simulink library "Brakes_ABS_4_Channel"  (R2019b)
settings: Solver=VariableStepAuto  StartTime=0.0  StopTime=10.0  RelTol=1e-3
undefined symbols (not defined in the file): Brakes
libraries: fl_lib x31, nesl_utility x18, sh_lib x9, sdl_lib x4, sm_car_lib x4
(part 1 of 2)
Description:
  | Component of Simscape Vehicle Templates Library
  | 
  | Copyright 2018-2020 The MathWorks, Inc.
settings Model: Creator=smiller  LastModifiedBy=smiller
settings DataIOCC: ReturnWorkspaceOutputs=off
settings DebuggingCC: ArithmeticOperatorsInVariantConditions=warning
settings SFSimCC: CustomCodeUndefinedFunction=UseInterfaceOnly

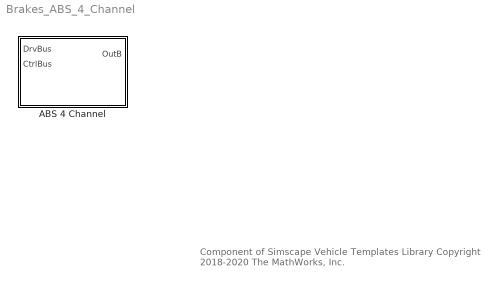
== system Brakes_ABS_4_Channel ==
  note: Component of Simscape Vehicle Templates Library
      | Copyright 2018-2020 The MathWorks, Inc.
  ABS 4 Channel : Subsystem  Tag=PublishSubsystem  VariantControl=ABS_4_Channel  mask(Four Channel ABS){d_caliper_bore_f=Brakes.Front.Caliper.lCylinderDiameter.Value, d_caliper_bore_r=Brakes.Rear.Caliper.lCylinderDiameter.Value, brk_pad_rad_fa=Brakes.Front.DiscAndPad.lMeanRadius.Value, brk_pad_rad_ra=Brakes.Rear.DiscAndPad.lMeanRadius.Value, brk_cyl_bore_fa=Brakes.Front.Caliper.lCylinderDiameter.Value, brk_cyl_bore_ra=Brakes.Rear.Caliper.lCylinderDiameter.Value, brk_n_pads_fa=Brakes.Front.DiscAndPad.NPads.Value, brk_n_pads_ra=Brakes.Rear.DiscAndPad.NPads.Value, brk_mu_static_fa=Brakes.Front.DiscAndPad.rMuStatic.Value, brk_mu_static_ra=Brakes.Rear.DiscAndPad.rMuStatic.Value, brk_mu_kin_fa=Brakes.Front.DiscAndPad.rMuKinetic.Value, brk_mu_kin_ra=Brakes.Rear.DiscAndPad.rMuKinetic.Value, brk_trans_vel_fa=Brakes.Front.DiscAndPad.nTransition.Value, brk_trans_vel_ra=Brakes.Rear.DiscAndPad.nTransition.Value, brk_visc_coef_fa=Brakes.Front.DiscAndPad.dViscous.Value, brk_visc_coef_ra=Brakes.Rear.DiscAndPad.dViscous.Value, spr_rate=Brakes.Front.ValveApply.kSpring.Value, D=Brakes.Front.ValveApply.bDamper.Value, area_max_apply=Brakes.Front.ValveApply.AMax.Value, open_max_apply=Brakes.Front.ValveApply.xMax.Value, area_max_rel=Brakes.Front.ValveRelease.AMax.Value, open_max_rel=Brakes.Front.ValveRelease.xMax.Value, p_max_f=Brakes.Front.Caliper.pMax.Value, p_max_r=Brakes.Rear.Caliper.pMax.Value, brkTs=Brakes.Front.ValveApply.fValveTime.Value}
      mask prompts: spr_rate "Spring Rate (N/m)"; D "Damping coefficient"; area_max_apply "Max Area Apply Valve (m^2)"; open_max_apply "Max Opening Apply Valve (m)"; area_max_rel "Max Area Release Valve (m^2)"; open_max_rel "Max Opening Release Valve (m)"; p_max_f "Max Master Cylinder Pressure Front (bar)"; p_max_r "Max Master Cylinder Pressure Rear (bar)"; brkTs "Filter time constant"
      mask init:
      | pist_area_pist_f = pi*d_caliper_bore_f^2/4;
      | pist_area_pist_r = pi*d_caliper_bore_r^2/4;
      mask TypeOptions brk_pad_rad_fa:
      | Disc
      | Brake
      | FL/r_mean | Disc
      | Brake
      | FR/r_mean
      mask TypeOptions brk_pad_rad_ra:
      | Disc
      | Brake
      | RL/r_mean | Disc
      | Brake
      | RR/r_mean
      mask TypeOptions brk_cyl_bore_fa:
      | Disc
      | Brake
      | FL/bore | Disc
      | Brake
      | FR/bore
      mask TypeOptions brk_cyl_bore_ra:
      | Disc
      | Brake
      | RL/bore | Disc
      | Brake
      | RR/bore
      mask TypeOptions brk_n_pads_fa:
      | Disc
      | Brake
      | FL/n_pads | Disc
      | Brake
      | FR/n_pads
      mask TypeOptions brk_n_pads_ra:
      | Disc
      | Brake
      | RL/n_pads | Disc
      | Brake
      | RR/n_pads
      mask TypeOptions brk_mu_static_fa:
      | Disc
      | Brake
      | FL/mu_static | Disc
      | Brake
      | FR/mu_static
      mask TypeOptions brk_mu_static_ra:
      | Disc
      | Brake
      | RL/mu_static | Disc
      | Brake
      | RR/mu_static
      mask TypeOptions brk_mu_kin_fa:
      | Disc
      | Brake
      | FL/mu_coulomb | Disc
      | Brake
      | FR/mu_coulomb
      mask TypeOptions brk_mu_kin_ra:
      | Disc
      | Brake
      | RL/mu_coulomb | Disc
      | Brake
      | RR/mu_coulomb
      mask TypeOptions brk_trans_vel_fa:
      | Disc
      | Brake
      | FL/brkwy_vel | Disc
      | Brake
      | FR/brkwy_vel
      mask TypeOptions brk_trans_vel_ra:
      | Disc
      | Brake
      | RL/brkwy_vel | Disc
      | Brake
      | RR/brkwy_vel
      mask TypeOptions brk_visc_coef_fa:
      | Disc
      | Brake
      | FL/visc_coef
      mask TypeOptions brk_visc_coef_ra:
      | Disc
      | Brake
      | RL/visc_coef | Disc
      | Brake
      | RR/visc_coef
      mask TypeOptions spr_rate: Valves/spr_rate
      mask TypeOptions D: Valves/D
      mask TypeOptions area_max_apply: Valves/area_max_apply
      mask TypeOptions open_max_apply: Valves/open_max_apply
      mask TypeOptions area_max_rel: Valves/area_max_rel
      mask TypeOptions open_max_rel: Valves/open_max_rel
      mask TypeOptions p_max_f: Valves/p_max_f
      mask TypeOptions p_max_r: Valves/p_max_r
      mask TypeOptions brkTs: Valves/brkTs
      mask DialogControl Container10 Prompt: Geometry
      mask DialogControl cont_brk_geom Prompt: Geometry
      mask DialogControl text_brakes_fa Prompt: Front Susp.
      mask DialogControl text_brakes_ra Prompt: Rear Susp.
      mask DialogControl text_caliper_bore Prompt: Caliper Bore (m)
      mask DialogControl text_brakes_pad_rad Prompt: Mean Pad Radius (m)
      mask DialogControl text_brakes_cyl_bore Prompt: Cylinder Bore (m)
      mask DialogControl text_brakes_n_pads Prompt: Number of pads
      mask DialogControl Container9 Prompt: Friction
      mask DialogControl cont_brk_frict Prompt: Friction
      mask DialogControl text_brakes_mu_static Prompt: Static Coeff. (0-1)
      mask DialogControl text_brakes_mu_kin Prompt: Kinetic Coeff. (0-1)
      mask DialogControl text_brakes_trans_vel Prompt: Trans. Velocity (rad/s)
      mask DialogControl text_brakes_visc_coef Prompt: Viscous (N*m/(rad/s))
      mask DialogControl cont_valves Prompt: Valves
      mask Display: image('sm_car_vehicle_brakes_abs_IMAGE.png');

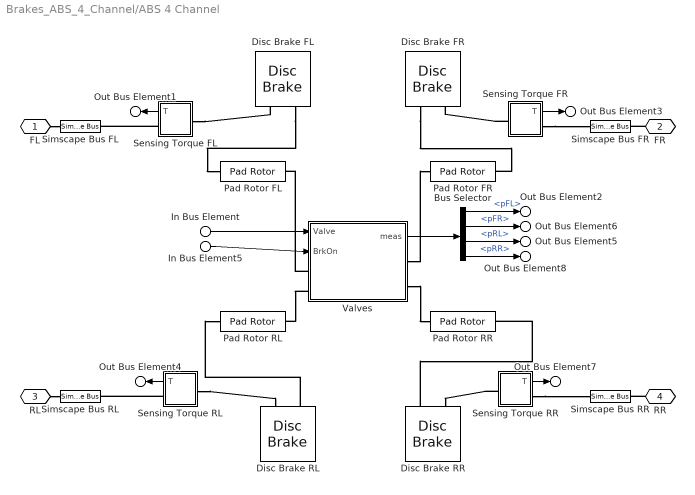
== system Brakes_ABS_4_Channel/ABS 4 Channel ==
  In Bus Element5 : Inport  PortName=DrvBus  Element=rBrakePedal
  In Bus Element : Inport  Port=2  PortName=CtrlBus  Element=Valves
  Bus Selector : BusSelector  OutputSignals=pFL,pFR,pRL,pRR
  Disc Brake FL : sdl_lib/Brakes & Detents/Rotational/Disc Brake  r_mean=brk_pad_rad_fa m  bore=brk_cyl_bore_fa m  n_pads=brk_n_pads_fa  thermal_port=simscape.enum.thermaleffects.omit  mu_static=brk_mu_static_fa  mu_coulomb=brk_mu_kin_fa  temperature_TLU=[280, 300, 320] K  mu_static_TLU=[.9, .8, .7]  mu_coulomb_TLU=[.8, .7, .6]  thermal_mass=50 kJ/K  brkwy_vel=brk_trans_vel_fa rad/s  visc_coef=brk_visc_coef_fa N*m/(rad/s)  temperature_specify=off  temperature_priority=High  temperature=300 K  temperature_nominal_specify=off  temperature_nominal_unit=K  temperature_nominal_value=1
      settings: SourceProductName=Simscape Driveline  SourceProductBaseCode=LD
  Disc Brake FR : sdl_lib/Brakes & Detents/Rotational/Disc Brake  r_mean=brk_pad_rad_fa m  bore=brk_cyl_bore_fa m  n_pads=brk_n_pads_fa  thermal_port=simscape.enum.thermaleffects.omit  mu_static=brk_mu_static_fa  mu_coulomb=brk_mu_kin_fa  temperature_TLU=[280, 300, 320] K  mu_static_TLU=[.9, .8, .7]  mu_coulomb_TLU=[.8, .7, .6]  thermal_mass=50 kJ/K  brkwy_vel=brk_trans_vel_fa rad/s  visc_coef=.001 N*m/(rad/s)  temperature_specify=off  temperature_priority=High  temperature=300 K  temperature_nominal_specify=off  temperature_nominal_unit=K  temperature_nominal_value=1
      settings: SourceProductName=Simscape Driveline  SourceProductBaseCode=LD
  Disc Brake RL : sdl_lib/Brakes & Detents/Rotational/Disc Brake  r_mean=brk_pad_rad_ra m  bore=brk_cyl_bore_ra m  n_pads=brk_n_pads_ra  thermal_port=simscape.enum.thermaleffects.omit  mu_static=brk_mu_static_ra  mu_coulomb=brk_mu_kin_ra  temperature_TLU=[280, 300, 320] K  mu_static_TLU=[.9, .8, .7]  mu_coulomb_TLU=[.8, .7, .6]  thermal_mass=50 kJ/K  brkwy_vel=brk_trans_vel_ra rad/s  visc_coef=brk_visc_coef_ra N*m/(rad/s)  temperature_specify=off  temperature_priority=High  temperature=300 K  temperature_nominal_specify=off  temperature_nominal_unit=K  temperature_nominal_value=1
      settings: SourceProductName=Simscape Driveline  SourceProductBaseCode=LD
  Disc Brake RR : sdl_lib/Brakes & Detents/Rotational/Disc Brake  r_mean=brk_pad_rad_ra m  bore=brk_cyl_bore_ra m  n_pads=brk_n_pads_ra  thermal_port=simscape.enum.thermaleffects.omit  mu_static=brk_mu_static_ra  mu_coulomb=brk_mu_kin_ra  temperature_TLU=[280, 300, 320] K  mu_static_TLU=[.9, .8, .7]  mu_coulomb_TLU=[.8, .7, .6]  thermal_mass=50 kJ/K  brkwy_vel=brk_trans_vel_ra rad/s  visc_coef=brk_visc_coef_ra N*m/(rad/s)  temperature_specify=off  temperature_priority=High  temperature=300 K  temperature_nominal_specify=off  temperature_nominal_unit=K  temperature_nominal_value=1
      settings: SourceProductName=Simscape Driveline  SourceProductBaseCode=LD
  Pad Rotor FL : sm_car_lib/Brakes/Pad Rotor  d_caliper_piston_f=d_caliper_bore_f
  Pad Rotor FR : sm_car_lib/Brakes/Pad Rotor  d_caliper_piston_f=d_caliper_bore_f
  Pad Rotor RL : sm_car_lib/Brakes/Pad Rotor  d_caliper_piston_f=d_caliper_bore_r
  Pad Rotor RR : sm_car_lib/Brakes/Pad Rotor  d_caliper_piston_f=d_caliper_bore_r
  Sensing Torque FL : Subsystem
  Sensing Torque FR : Subsystem
  Sensing Torque RL : Subsystem
  Sensing Torque RR : Subsystem
  Simscape Bus FL : SimscapeBus  HierarchyStrings=Axle1D
  Simscape Bus FR : SimscapeBus  HierarchyStrings=Axle1D
  Simscape Bus RL : SimscapeBus  HierarchyStrings=Axle1D
  Simscape Bus RR : SimscapeBus  HierarchyStrings=Axle1D
  Valves : Subsystem  VariantControl=Valves  mask{brkTs=brkTs, p_max_f=p_max_f, p_max_r=p_max_r, spr_rate=spr_rate, D=D, area_max_apply=area_max_apply, open_max_apply=open_max_apply, area_max_rel=area_max_rel, open_max_rel=open_max_rel}
      mask prompts: brkTs "Filter time constant"; p_max_f "Max Pressure Front (bar)"; p_max_r "Max Pressure Rear (bar)"; spr_rate "Spring Rate (N/m)"; D "Damping coefficient"; area_max_apply "Max Area Apply Valve (m^2)"; open_max_apply "Max Opening Apply Valve (m)"; area_max_rel "Max Area Release Valve (m^2)"; open_max_rel "Max Opening Release Valve (m)"
      mask TypeOptions brkTs:
      | Valves FL/Actuator
      | Dynamics/b | Valves FR/Actuator
      | Dynamics/b | Valves RL/Actuator
      | Dynamics/b | Valves RR/Actuator
      | Dynamics/b
      mask TypeOptions p_max_f: MC Pressure F/Value
      mask TypeOptions p_max_r: MC Pressure R/Value
      mask TypeOptions spr_rate: Return Spring FL/Spring/spr_rate | Return Spring FR/Spring/spr_rate | Return Spring RL/Spring/spr_rate | Return Spring RR/Spring/spr_rate
      mask TypeOptions D: Return Spring FL/Damper/D | Return Spring FR/Damper/D | Return Spring RL/Damper/D | Return Spring RR/Damper/D
  FL : PMIOPort  Side=Left
  FR : PMIOPort  Port=2  Side=Right
  RL : PMIOPort  Port=3  Side=Left
  RR : PMIOPort  Port=4  Side=Right
  Out Bus Element1 : Outport  VectorParamsAs1DForOutWhenUnconnected=off  PortName=OutB  Element=MBrakeFL
  Out Bus Element3 : Outport  VectorParamsAs1DForOutWhenUnconnected=off  PortName=OutB  Element=MBrakeFR
  Out Bus Element4 : Outport  VectorParamsAs1DForOutWhenUnconnected=off  PortName=OutB  Element=MBrakeRL
  Out Bus Element7 : Outport  VectorParamsAs1DForOutWhenUnconnected=off  PortName=OutB  Element=MBrakeRR
  Out Bus Element2 : Outport  VectorParamsAs1DForOutWhenUnconnected=off  PortName=OutB  Element=pBrakeFL
  Out Bus Element6 : Outport  VectorParamsAs1DForOutWhenUnconnected=off  PortName=OutB  Element=pBrakeFR
  Out Bus Element5 : Outport  VectorParamsAs1DForOutWhenUnconnected=off  PortName=OutB  Element=pBrakeRL
  Out Bus Element8 : Outport  VectorParamsAs1DForOutWhenUnconnected=off  PortName=OutB  Element=pBrakeRR
  wires:
  Sensing Torque FL/1(T) -> Out Bus Element1/1
  Bus Selector/4 -> Out Bus Element8/1  "<pRR>"
  Sensing Torque FR/1(T) -> Out Bus Element3/1
  Sensing Torque RR/1(T) -> Out Bus Element7/1
  Bus Selector/2 -> Out Bus Element6/1  "<pFR>"
  Bus Selector/1 -> Out Bus Element2/1  "<pFL>"
  Sensing Torque RL/1(T) -> Out Bus Element4/1
  Bus Selector/3 -> Out Bus Element5/1  "<pRL>"
  Valves/1(meas) -> Bus Selector/1
  In Bus Element/1 -> Valves/1(Valve)
  In Bus Element5/1 -> Valves/2(BrkOn)
  connections:
  Sensing Torque RL/RConn1 -- Simscape Bus RL/LConn1
  Valves/LConn2 -- Pad Rotor RL/RConn1
  Disc Brake FR/LConn1 -- Pad Rotor FR/LConn1
  Sensing Torque FR/LConn1 -- Disc Brake FR/LConn2
  Disc Brake RR/LConn1 -- Pad Rotor RR/LConn1
  Valves/RConn2 -- Pad Rotor RR/RConn1
  RL/RConn1 -- Simscape Bus RL/RConn1
  Sensing Torque RR/LConn1 -- Disc Brake RR/LConn2
  Sensing Torque FR/RConn1 -- Simscape Bus FR/LConn1
  Disc Brake RL/LConn1 -- Pad Rotor RL/LConn1
  Sensing Torque RR/RConn1 -- Simscape Bus RR/LConn1
  Sensing Torque FL/RConn1 -- Simscape Bus FL/LConn1
  Sensing Torque FL/LConn1 -- Disc Brake FL/LConn2
  RR/RConn1 -- Simscape Bus RR/RConn1
  FR/RConn1 -- Simscape Bus FR/RConn1
  Sensing Torque RL/LConn1 -- Disc Brake RL/LConn2
  Valves/LConn1 -- Pad Rotor FL/RConn1
  Disc Brake FL/LConn1 -- Pad Rotor FL/LConn1
  FL/RConn1 -- Simscape Bus FL/RConn1
  Valves/RConn1 -- Pad Rotor FR/RConn1

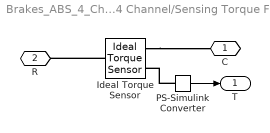
== system Brakes_ABS_4_Channel/ABS 4 Channel/Sensing Torque FL ==
  Ideal Torque Sensor : fl_lib/Mechanical/Mechanical Sensors/Ideal Torque Sensor
  PS-Simulink Converter : nesl_utility/PS-Simulink Converter  PhysicalDomain=network_engine_domain  SubClassName=ps_output  LeftPortType=input  RightPortType=output  PseudoPeriodic=off  Frequencies=[]  Unit=N*m  AffineConversion=off
  C : PMIOPort  Side=Right
  R : PMIOPort  Port=2  Side=Left
  T : Outport  VectorParamsAs1DForOutWhenUnconnected=off
  wires:
  PS-Simulink Converter/1 -> T/1
  connections:
  Ideal Torque Sensor/LConn1 -- R/RConn1
  Ideal Torque Sensor/RConn1 -- C/RConn1
  PS-Simulink Converter/LConn1 -- Ideal Torque Sensor/RConn2

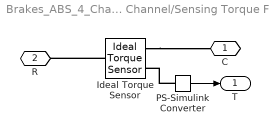
== system Brakes_ABS_4_Channel/ABS 4 Channel/Sensing Torque FR ==
  Ideal Torque Sensor : fl_lib/Mechanical/Mechanical Sensors/Ideal Torque Sensor
  PS-Simulink Converter : nesl_utility/PS-Simulink Converter  PhysicalDomain=network_engine_domain  SubClassName=ps_output  LeftPortType=input  RightPortType=output  PseudoPeriodic=off  Frequencies=[]  Unit=N*m  AffineConversion=off
  C : PMIOPort  Side=Right
  R : PMIOPort  Port=2  Side=Left
  T : Outport  VectorParamsAs1DForOutWhenUnconnected=off
  wires:
  PS-Simulink Converter/1 -> T/1
  connections:
  Ideal Torque Sensor/LConn1 -- R/RConn1
  Ideal Torque Sensor/RConn1 -- C/RConn1
  PS-Simulink Converter/LConn1 -- Ideal Torque Sensor/RConn2

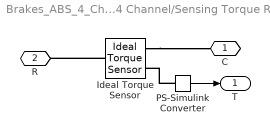
== system Brakes_ABS_4_Channel/ABS 4 Channel/Sensing Torque RL ==
  Ideal Torque Sensor : fl_lib/Mechanical/Mechanical Sensors/Ideal Torque Sensor
  PS-Simulink Converter : nesl_utility/PS-Simulink Converter  PhysicalDomain=network_engine_domain  SubClassName=ps_output  LeftPortType=input  RightPortType=output  PseudoPeriodic=off  Frequencies=[]  Unit=N*m  AffineConversion=off
  C : PMIOPort  Side=Right
  R : PMIOPort  Port=2  Side=Left
  T : Outport  VectorParamsAs1DForOutWhenUnconnected=off
  wires:
  PS-Simulink Converter/1 -> T/1
  connections:
  PS-Simulink Converter/LConn1 -- Ideal Torque Sensor/RConn2
  Ideal Torque Sensor/RConn1 -- C/RConn1
  Ideal Torque Sensor/LConn1 -- R/RConn1

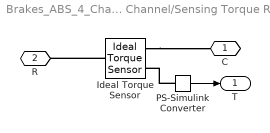
== system Brakes_ABS_4_Channel/ABS 4 Channel/Sensing Torque RR ==
  Ideal Torque Sensor : fl_lib/Mechanical/Mechanical Sensors/Ideal Torque Sensor
  PS-Simulink Converter : nesl_utility/PS-Simulink Converter  PhysicalDomain=network_engine_domain  SubClassName=ps_output  LeftPortType=input  RightPortType=output  PseudoPeriodic=off  Frequencies=[]  Unit=N*m  AffineConversion=off
  C : PMIOPort  Side=Right
  R : PMIOPort  Port=2  Side=Left
  T : Outport  VectorParamsAs1DForOutWhenUnconnected=off
  wires:
  PS-Simulink Converter/1 -> T/1
  connections:
  PS-Simulink Converter/LConn1 -- Ideal Torque Sensor/RConn2
  Ideal Torque Sensor/RConn1 -- C/RConn1
  Ideal Torque Sensor/LConn1 -- R/RConn1

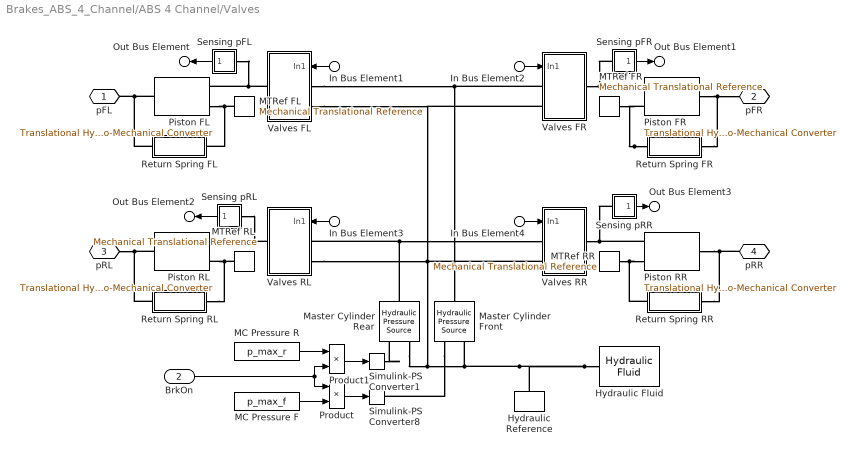
== system Brakes_ABS_4_Channel/ABS 4 Channel/Valves ==
  In Bus Element1 : Inport  PortName=Valve  Element=FL
  In Bus Element2 : Inport  PortName=Valve  Element=FR
  In Bus Element3 : Inport  PortName=Valve  Element=RL
  In Bus Element4 : Inport  PortName=Valve  Element=RR
  BrkOn : Inport  Port=2
  Hydraulic Fluid : sh_lib/Hydraulic Utilities/Hydraulic Fluid  DataSource=1  SelFluid=17  SysTemp=60  TrapAir=0.005  ViscDerFactor=1  range_error=2
      settings: SourceProductName=Simscape Fluids
  Hydraulic Reference : fl_lib/Hydraulic/Hydraulic Elements/Hydraulic Reference
      settings: SourceProductName=Simscape
  MC Pressure F : Constant  Value=p_max_f
  MC Pressure R : Constant  Value=p_max_r
  MTRef FL : fl_lib/Mechanical/Translational Elements/Mechanical Translational Reference
  MTRef FR : fl_lib/Mechanical/Translational Elements/Mechanical Translational Reference
  MTRef RL : fl_lib/Mechanical/Translational Elements/Mechanical Translational Reference
  MTRef RR : fl_lib/Mechanical/Translational Elements/Mechanical Translational Reference
  Master Cylinder Front : fl_lib/Hydraulic/Hydraulic Sources/Hydraulic Pressure Source
      settings: SourceProductName=Simscape  SourceProductBaseCode=SS  InternalSimscapePortConfiguration="{\"Bottom\":[],\"Left\":[{\"id\":\"P\",\"label\":\"P\",\"type\":\"foundation.hydraulic.hydraulic\"}],\"Right\":[{\"id\":\"S\",\"label\":\"S\",\"type\":\"input\"},{\"id\":\"T\",\"label\":\"T\",\"type\":\"foundation.hydraulic.hydraulic\"}],\"Top\":[]}"
  Master Cylinder Rear : fl_lib/Hydraulic/Hydraulic Sources/Hydraulic Pressure Source
      settings: SourceProductName=Simscape  SourceProductBaseCode=SS  InternalSimscapePortConfiguration="{\"Bottom\":[],\"Left\":[{\"id\":\"P\",\"label\":\"P\",\"type\":\"foundation.hydraulic.hydraulic\"}],\"Right\":[{\"id\":\"S\",\"label\":\"S\",\"type\":\"input\"},{\"id\":\"T\",\"label\":\"T\",\"type\":\"foundation.hydraulic.hydraulic\"}],\"Top\":[]}"
  Piston FL : fl_lib/Hydraulic/Hydraulic Elements/Translational Hydro-Mechanical Converter  area=pist_area_pist_f m^2  or=1  compressibility=1  init_pos=0 m  V_dead=1e-4 m^3  k_sh=1.4  initial_pressure=0 Pa
      settings: SourceProductName=Simscape  SourceProductBaseCode=SS  InternalSimscapePortConfiguration="{\"Bottom\":[],\"Left\":[{\"id\":\"C\",\"label\":\"C\",\"type\":\"foundation.mechanical.translational.translational\"},{\"id\":\"A\",\"label\":\"A\",\"type\":\"foundation.hydraulic.hydraulic\"}],\"Right\":[{\"id\":\"R\",\"label\":\"R\",\"type\":\"foundation.mechanical.translational.translational\"}],\"Top\":[]}"
  Piston FR : fl_lib/Hydraulic/Hydraulic Elements/Translational Hydro-Mechanical Converter  area=pist_area_pist_f m^2  or=1  compressibility=1  init_pos=0 m  V_dead=1e-4 m^3  k_sh=1.4  initial_pressure=0 Pa
      settings: SourceProductName=Simscape  SourceProductBaseCode=SS  InternalSimscapePortConfiguration="{\"Bottom\":[],\"Left\":[{\"id\":\"C\",\"label\":\"C\",\"type\":\"foundation.mechanical.translational.translational\"},{\"id\":\"A\",\"label\":\"A\",\"type\":\"foundation.hydraulic.hydraulic\"}],\"Right\":[{\"id\":\"R\",\"label\":\"R\",\"type\":\"foundation.mechanical.translational.translational\"}],\"Top\":[]}"
  Piston RL : fl_lib/Hydraulic/Hydraulic Elements/Translational Hydro-Mechanical Converter  area=pist_area_pist_r m^2  or=1  compressibility=1  init_pos=0 m  V_dead=1e-4 m^3  k_sh=1.4  initial_pressure=0 Pa
      settings: SourceProductName=Simscape  SourceProductBaseCode=SS  InternalSimscapePortConfiguration="{\"Bottom\":[],\"Left\":[{\"id\":\"C\",\"label\":\"C\",\"type\":\"foundation.mechanical.translational.translational\"},{\"id\":\"A\",\"label\":\"A\",\"type\":\"foundation.hydraulic.hydraulic\"}],\"Right\":[{\"id\":\"R\",\"label\":\"R\",\"type\":\"foundation.mechanical.translational.translational\"}],\"Top\":[]}"
  Piston RR : fl_lib/Hydraulic/Hydraulic Elements/Translational Hydro-Mechanical Converter  area=pist_area_pist_r m^2  or=1  compressibility=1  init_pos=0 m  V_dead=1e-4 m^3  k_sh=1.4  initial_pressure=0 Pa
      settings: SourceProductName=Simscape  SourceProductBaseCode=SS  InternalSimscapePortConfiguration="{\"Bottom\":[],\"Left\":[{\"id\":\"C\",\"label\":\"C\",\"type\":\"foundation.mechanical.translational.translational\"},{\"id\":\"A\",\"label\":\"A\",\"type\":\"foundation.hydraulic.hydraulic\"}],\"Right\":[{\"id\":\"R\",\"label\":\"R\",\"type\":\"foundation.mechanical.translational.translational\"}],\"Top\":[]}"
  Product : Product
  Product1 : Product
  Return Spring FL : Subsystem
  Return Spring FR : Subsystem
  Return Spring RL : Subsystem
  Return Spring RR : Subsystem
  Sensing pFL : Subsystem
  Sensing pFR : Subsystem
  Sensing pRL : Subsystem
  Sensing pRR : Subsystem
  Simulink-PS Converter1 : nesl_utility/Simulink-PS Converter  PhysicalDomain=network_engine_domain  SubClassName=ps_input  LeftPortType=input  RightPortType=output  PseudoPeriodic=off  Frequencies=[]  NoiseDistribution=none  NoiseParameters=[]  Unit=bar  AffineConversion=off  FilteringAndDerivatives=provide  SimscapeFilterOrder=1  InputFilterTimeConstant=0.001  UdotUserProvided=0
  Simulink-PS Converter8 : nesl_utility/Simulink-PS Converter  PhysicalDomain=network_engine_domain  SubClassName=ps_input  LeftPortType=input  RightPortType=output  PseudoPeriodic=off  Frequencies=[]  NoiseDistribution=none  NoiseParameters=[]  Unit=bar  AffineConversion=off  FilteringAndDerivatives=provide  SimscapeFilterOrder=1  InputFilterTimeConstant=0.001  UdotUserProvided=0
  Valves FL : Subsystem
  Valves FR : Subsystem
  Valves RL : Subsystem
  Valves RR : Subsystem
  pFL : PMIOPort  Side=Left
  pFR : PMIOPort  Port=2  Side=Right
  pRL : PMIOPort  Port=3  Side=Left
  pRR : PMIOPort  Port=4  Side=Right
  Out Bus Element : Outport  VectorParamsAs1DForOutWhenUnconnected=off  PortName=meas  Element=pFL
  Out Bus Element1 : Outport  VectorParamsAs1DForOutWhenUnconnected=off  PortName=meas  Element=pFR
  Out Bus Element2 : Outport  VectorParamsAs1DForOutWhenUnconnected=off  PortName=meas  Element=pRL
  Out Bus Element3 : Outport  VectorParamsAs1DForOutWhenUnconnected=off  PortName=meas  Element=pRR
  wires:
  Product/1 -> Simulink-PS Converter8/1
  BrkOn/1 -> Product/1, Product1/2
  In Bus Element3/1 -> Valves RL/1(In1)
  In Bus Element4/1 -> Valves RR/1(In1)
  In Bus Element2/1 -> Valves FR/1(In1)
  In Bus Element1/1 -> Valves FL/1(In1)
  MC Pressure F/1 -> Product/2
  Sensing pRL/1(p) -> Out Bus Element2/1
  Sensing pRR/1(p) -> Out Bus Element3/1
  Sensing pFR/1(p) -> Out Bus Element1/1
  Sensing pFL/1(p) -> Out Bus Element/1
  Product1/1 -> Simulink-PS Converter1/1
  MC Pressure R/1 -> Product1/1
  connections:
  Return Spring FR/LConn1 -- MTRef FR/LConn1 -- Piston FR/LConn1
  MTRef FL/LConn1 -- Return Spring FL/LConn1 -- Piston FL/LConn1
  MTRef RL/LConn1 -- Piston RL/LConn1 -- Return Spring RL/LConn1
  Sensing pFL/LConn1 -- Piston FL/LConn2 -- Valves FL/RConn1
  Master Cylinder Front/RConn1 -- Simulink-PS Converter8/RConn1
  Valves FR/LConn1 -- Valves FL/LConn1 -- Master Cylinder Front/LConn1
  Hydraulic Fluid/RConn1 -- Master Cylinder Rear/RConn2 -- Valves RR/LConn2 -- Valves FR/LConn2 -- Valves FL/LConn2 -- Valves RL/LConn2 -- Master Cylinder Front/RConn2 -- Hydraulic Reference/LConn1
  Return Spring RL/RConn1 -- pRL/RConn1 -- Piston RL/RConn1
  Return Spring RR/RConn1 -- pRR/RConn1 -- Piston RR/RConn1
  Piston FR/RConn1 -- pFR/RConn1 -- Return Spring FR/RConn1
  Piston FL/RConn1 -- Return Spring FL/RConn1 -- pFL/RConn1
  Piston RR/LConn1 -- MTRef RR/LConn1 -- Return Spring RR/LConn1
  Sensing pRL/LConn1 -- Valves RL/RConn1 -- Piston RL/LConn2
  Sensing pRR/LConn1 -- Valves RR/RConn1 -- Piston RR/LConn2
  Sensing pFR/LConn1 -- Valves FR/RConn1 -- Piston FR/LConn2
  Simulink-PS Converter1/RConn1 -- Master Cylinder Rear/RConn1
  Master Cylinder Rear/LConn1 -- Valves RR/LConn1 -- Valves RL/LConn1

== system Brakes_ABS_4_Channel/ABS 4 Channel/Valves/Return Spring FL ==
  Damper : fl_lib/Mechanical/Translational Elements/Translational Damper  D=D N/(m/s)  v_specify=off  v_priority=None  v=0 m/s  v_nominal_specify=off  v_nominal_unit=m/s  v_nominal_value=1  f_specify=off  f_priority=None  f=0 N  f_nominal_specify=off  f_nominal_unit=N  f_nominal_value=1
  Spring : fl_lib/Mechanical/Translational Elements/Translational Spring  spr_rate=spr_rate N/m  v_specify=off  v_priority=None  v=0 m/s  v_nominal_specify=off  v_nominal_unit=m/s  v_nominal_value=1  f_specify=off  f_priority=None  f=0 N  f_nominal_specify=off  f_nominal_unit=N  f_nominal_value=1  x_specify=off  x_priority=High  x=0 m  x_nominal_specify=off  x_nominal_unit=m  x_nominal_value=1
  R : PMIOPort  Side=Right
  C : PMIOPort  Port=2  Side=Left
  connections:
  Spring/RConn1 -- Damper/RConn1 -- C/RConn1
  Spring/LConn1 -- R/RConn1 -- Damper/LConn1

== system Brakes_ABS_4_Channel/ABS 4 Channel/Valves/Return Spring FR ==
  Damper : fl_lib/Mechanical/Translational Elements/Translational Damper  D=D N/(m/s)  v_specify=off  v_priority=None  v=0 m/s  v_nominal_specify=off  v_nominal_unit=m/s  v_nominal_value=1  f_specify=off  f_priority=None  f=0 N  f_nominal_specify=off  f_nominal_unit=N  f_nominal_value=1
  Spring : fl_lib/Mechanical/Translational Elements/Translational Spring  spr_rate=spr_rate N/m  v_specify=off  v_priority=None  v=0 m/s  v_nominal_specify=off  v_nominal_unit=m/s  v_nominal_value=1  f_specify=off  f_priority=None  f=0 N  f_nominal_specify=off  f_nominal_unit=N  f_nominal_value=1  x_specify=off  x_priority=High  x=0 m  x_nominal_specify=off  x_nominal_unit=m  x_nominal_value=1
  R : PMIOPort  Side=Right
  C : PMIOPort  Port=2  Side=Left
  connections:
  Damper/LConn1 -- R/RConn1 -- Spring/LConn1
  C/RConn1 -- Damper/RConn1 -- Spring/RConn1

== system Brakes_ABS_4_Channel/ABS 4 Channel/Valves/Return Spring RL ==
  Damper : fl_lib/Mechanical/Translational Elements/Translational Damper  D=D N/(m/s)  v_specify=off  v_priority=None  v=0 m/s  v_nominal_specify=off  v_nominal_unit=m/s  v_nominal_value=1  f_specify=off  f_priority=None  f=0 N  f_nominal_specify=off  f_nominal_unit=N  f_nominal_value=1
  Spring : fl_lib/Mechanical/Translational Elements/Translational Spring  spr_rate=spr_rate N/m  v_specify=off  v_priority=None  v=0 m/s  v_nominal_specify=off  v_nominal_unit=m/s  v_nominal_value=1  f_specify=off  f_priority=None  f=0 N  f_nominal_specify=off  f_nominal_unit=N  f_nominal_value=1  x_specify=off  x_priority=High  x=0 m  x_nominal_specify=off  x_nominal_unit=m  x_nominal_value=1
  R : PMIOPort  Side=Right
  C : PMIOPort  Port=2  Side=Left
  connections:
  R/RConn1 -- Damper/LConn1 -- Spring/LConn1
  C/RConn1 -- Spring/RConn1 -- Damper/RConn1

== system Brakes_ABS_4_Channel/ABS 4 Channel/Valves/Return Spring RR ==
  Damper : fl_lib/Mechanical/Translational Elements/Translational Damper  D=D N/(m/s)  v_specify=off  v_priority=None  v=0 m/s  v_nominal_specify=off  v_nominal_unit=m/s  v_nominal_value=1  f_specify=off  f_priority=None  f=0 N  f_nominal_specify=off  f_nominal_unit=N  f_nominal_value=1
  Spring : fl_lib/Mechanical/Translational Elements/Translational Spring  spr_rate=spr_rate N/m  v_specify=off  v_priority=None  v=0 m/s  v_nominal_specify=off  v_nominal_unit=m/s  v_nominal_value=1  f_specify=off  f_priority=None  f=0 N  f_nominal_specify=off  f_nominal_unit=N  f_nominal_value=1  x_specify=off  x_priority=High  x=0 m  x_nominal_specify=off  x_nominal_unit=m  x_nominal_value=1
  R : PMIOPort  Side=Right
  C : PMIOPort  Port=2  Side=Left
  connections:
  Spring/RConn1 -- Damper/RConn1 -- C/RConn1
  Spring/LConn1 -- R/RConn1 -- Damper/LConn1

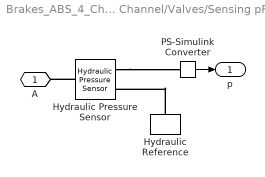
== system Brakes_ABS_4_Channel/ABS 4 Channel/Valves/Sensing pFL ==
  Hydraulic Pressure Sensor : fl_lib/Hydraulic/Hydraulic Sensors/Hydraulic Pressure Sensor
      settings: SourceProductName=Simscape
  Hydraulic Reference : fl_lib/Hydraulic/Hydraulic Elements/Hydraulic Reference
      settings: SourceProductName=Simscape
  PS-Simulink Converter : nesl_utility/PS-Simulink Converter  PhysicalDomain=network_engine_domain  SubClassName=ps_output  LeftPortType=input  RightPortType=output  PseudoPeriodic=off  Frequencies=[]  Unit=bar  AffineConversion=off
  A : PMIOPort  Side=Left
  p : Outport  VectorParamsAs1DForOutWhenUnconnected=off
  wires:
  PS-Simulink Converter/1 -> p/1
  connections:
  Hydraulic Reference/LConn1 -- Hydraulic Pressure Sensor/RConn1
  Hydraulic Pressure Sensor/LConn1 -- A/RConn1
  Hydraulic Pressure Sensor/RConn2 -- PS-Simulink Converter/LConn1

== system Brakes_ABS_4_Channel/ABS 4 Channel/Valves/Sensing pFR ==
  Hydraulic Pressure Sensor : fl_lib/Hydraulic/Hydraulic Sensors/Hydraulic Pressure Sensor
      settings: SourceProductName=Simscape
  Hydraulic Reference : fl_lib/Hydraulic/Hydraulic Elements/Hydraulic Reference
      settings: SourceProductName=Simscape
  PS-Simulink Converter : nesl_utility/PS-Simulink Converter  PhysicalDomain=network_engine_domain  SubClassName=ps_output  LeftPortType=input  RightPortType=output  PseudoPeriodic=off  Frequencies=[]  Unit=bar  AffineConversion=off
  A : PMIOPort  Side=Left
  p : Outport  VectorParamsAs1DForOutWhenUnconnected=off
  wires:
  PS-Simulink Converter/1 -> p/1
  connections:
  Hydraulic Pressure Sensor/RConn2 -- PS-Simulink Converter/LConn1
  Hydraulic Pressure Sensor/LConn1 -- A/RConn1
  Hydraulic Reference/LConn1 -- Hydraulic Pressure Sensor/RConn1

== system Brakes_ABS_4_Channel/ABS 4 Channel/Valves/Sensing pRL ==
  Hydraulic Pressure Sensor : fl_lib/Hydraulic/Hydraulic Sensors/Hydraulic Pressure Sensor
      settings: SourceProductName=Simscape
  Hydraulic Reference : fl_lib/Hydraulic/Hydraulic Elements/Hydraulic Reference
      settings: SourceProductName=Simscape
  PS-Simulink Converter : nesl_utility/PS-Simulink Converter  PhysicalDomain=network_engine_domain  SubClassName=ps_output  LeftPortType=input  RightPortType=output  PseudoPeriodic=off  Frequencies=[]  Unit=bar  AffineConversion=off
  A : PMIOPort  Side=Left
  p : Outport  VectorParamsAs1DForOutWhenUnconnected=off
  wires:
  PS-Simulink Converter/1 -> p/1
  connections:
  Hydraulic Pressure Sensor/RConn2 -- PS-Simulink Converter/LConn1
  Hydraulic Pressure Sensor/LConn1 -- A/RConn1
  Hydraulic Reference/LConn1 -- Hydraulic Pressure Sensor/RConn1

== system Brakes_ABS_4_Channel/ABS 4 Channel/Valves/Sensing pRR ==
  Hydraulic Pressure Sensor : fl_lib/Hydraulic/Hydraulic Sensors/Hydraulic Pressure Sensor
      settings: SourceProductName=Simscape
  Hydraulic Reference : fl_lib/Hydraulic/Hydraulic Elements/Hydraulic Reference
      settings: SourceProductName=Simscape
  PS-Simulink Converter : nesl_utility/PS-Simulink Converter  PhysicalDomain=network_engine_domain  SubClassName=ps_output  LeftPortType=input  RightPortType=output  PseudoPeriodic=off  Frequencies=[]  Unit=bar  AffineConversion=off
  A : PMIOPort  Side=Left
  p : Outport  VectorParamsAs1DForOutWhenUnconnected=off
  wires:
  PS-Simulink Converter/1 -> p/1
  connections:
  Hydraulic Reference/LConn1 -- Hydraulic Pressure Sensor/RConn1
  Hydraulic Pressure Sensor/LConn1 -- A/RConn1
  Hydraulic Pressure Sensor/RConn2 -- PS-Simulink Converter/LConn1

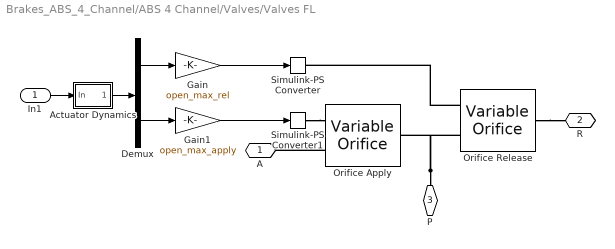
== system Brakes_ABS_4_Channel/ABS 4 Channel/Valves/Valves FL ==
  In1 : Inport
  Actuator Dynamics : Subsystem  mask(First-order lag supporting vector signals){b=brkTs, x_initial=0}
      mask prompts: b "Filter time constant"; x_initial "Initial output"
      mask help: Models a lag of the form 1/(b*s+1) where s is the Laplace operator.
  Demux : Demux  Outputs=2
  Gain : Gain  Gain=open_max_rel
      settings: AttributesFormatString=%<Gain>
  Gain1 : Gain  Gain=open_max_apply
      settings: AttributesFormatString=%<Gain>
  Orifice Apply : sh_lib/Orifices/Variable Orifice  mdl_type=1  area_max=area_max_apply m^2  opening_max=open_max_apply m  opening_tab=[-.002, 0, .002, .005, .015] m  area_tab=[1e-09, 2.0352e-07, 4.0736e-05, .00011438, .00034356] m^2  pressure_tab=[-10000000, -5000000, -2000000, 2000000, 5000000, 10000000] Pa  flow_rate_tab=[-1e-07, -7.0711e-08, -4.4721e-08, 4.4721e-08, 7.0711e-08, 1e-07; -2.0352e-05, -1.4391e-05, -9.1017e-06, 9.1017e-06, 1.4391e-05, 2.0352e-05; -.0040736, -.0028805, -.0018218, .0018218, .0028805, .0040736; -.011438, -.0080879, -.0051152, .0051152, .0080879, .011438; -.034356, -.024293, -.015364, .015364, .024293, .034356] m^3/s  interp_method=1  extrap_method=1  or=1  C_d=0.7  x_0=0 m  A_leak=1e-12 m^2  lam_spec=1  B_lam=0.999  Re_cr=12  flow_rate_specify=off  flow_rate_priority=None  flow_rate=0 m^3/s  flow_rate_nominal_specify=off  flow_rate_nominal_unit=m^3/s  flow_rate_nominal_value=1  pressure_drop_specify=off  pressure_drop_priority=None  pressure_drop=0 Pa  pressure_drop_nominal_specify=off  pressure_drop_nominal_unit=Pa  pressure_drop_nominal_value=1
      settings: SourceProductName=Simscape Fluids  SourceProductBaseCode=SH  InternalSimscapePortConfiguration="{\"Bottom\":[],\"Left\":[{\"id\":\"S\",\"label\":\"S\",\"type\":\"input\"},{\"id\":\"A\",\"label\":\"A\",\"type\":\"foundation.hydraulic.hydraulic\"}],\"Right\":[{\"id\":\"B\",\"label\":\"B\",\"type\":\"foundation.hydraulic.hydraulic\"}],\"Top\":[]}"
  Orifice Release : sh_lib/Orifices/Variable Orifice  mdl_type=1  area_max=area_max_rel m^2  opening_max=open_max_rel m  opening_tab=[-.002, 0, .002, .005, .015] m  area_tab=[1e-09, 2.0352e-07, 4.0736e-05, .00011438, .00034356] m^2  pressure_tab=[-10000000, -5000000, -2000000, 2000000, 5000000, 10000000] Pa  flow_rate_tab=[-1e-07, -7.0711e-08, -4.4721e-08, 4.4721e-08, 7.0711e-08, 1e-07; -2.0352e-05, -1.4391e-05, -9.1017e-06, 9.1017e-06, 1.4391e-05, 2.0352e-05; -.0040736, -.0028805, -.0018218, .0018218, .0028805, .0040736; -.011438, -.0080879, -.0051152, .0051152, .0080879, .011438; -.034356, -.024293, -.015364, .015364, .024293, .034356] m^3/s  interp_method=1  extrap_method=1  or=1  C_d=0.7  x_0=0 m  A_leak=1e-12 m^2  lam_spec=1  B_lam=0.999  Re_cr=12  flow_rate_specify=off  flow_rate_priority=None  flow_rate=0 m^3/s  flow_rate_nominal_specify=off  flow_rate_nominal_unit=m^3/s  flow_rate_nominal_value=1  pressure_drop_specify=off  pressure_drop_priority=None  pressure_drop=0 Pa  pressure_drop_nominal_specify=off  pressure_drop_nominal_unit=Pa  pressure_drop_nominal_value=1
      settings: SourceProductName=Simscape Fluids  SourceProductBaseCode=SH  InternalSimscapePortConfiguration="{\"Bottom\":[],\"Left\":[{\"id\":\"S\",\"label\":\"S\",\"type\":\"input\"},{\"id\":\"A\",\"label\":\"A\",\"type\":\"foundation.hydraulic.hydraulic\"}],\"Right\":[{\"id\":\"B\",\"label\":\"B\",\"type\":\"foundation.hydraulic.hydraulic\"}],\"Top\":[]}"
  Simulink-PS Converter : nesl_utility/Simulink-PS Converter  PhysicalDomain=network_engine_domain  SubClassName=ps_input  LeftPortType=input  RightPortType=output  PseudoPeriodic=off  Frequencies=[]  NoiseDistribution=none  NoiseParameters=[]  Unit=1  AffineConversion=off  FilteringAndDerivatives=provide  SimscapeFilterOrder=1  InputFilterTimeConstant=0.001  UdotUserProvided=0
  Simulink-PS Converter1 : nesl_utility/Simulink-PS Converter  PhysicalDomain=network_engine_domain  SubClassName=ps_input  LeftPortType=input  RightPortType=output  PseudoPeriodic=off  Frequencies=[]  NoiseDistribution=none  NoiseParameters=[]  Unit=1  AffineConversion=off  FilteringAndDerivatives=provide  SimscapeFilterOrder=1  InputFilterTimeConstant=0.001  UdotUserProvided=0
  A : PMIOPort  Side=Left
  R : PMIOPort  Port=2  Side=Left
  P : PMIOPort  Port=3  Side=Right
  wires:
  Actuator Dynamics/1(Out) -> Demux/1
  Demux/2 -> Gain1/1
  Demux/1 -> Gain/1
  In1/1 -> Actuator Dynamics/1(In)
  Gain/1 -> Simulink-PS Converter/1
  Gain1/1 -> Simulink-PS Converter1/1
  connections:
  Orifice Release/LConn1 -- Simulink-PS Converter/RConn1
  Orifice Apply/LConn2 -- A/RConn1
  Simulink-PS Converter1/RConn1 -- Orifice Apply/LConn1
  Orifice Release/RConn1 -- R/RConn1
  P/RConn1 -- Orifice Apply/RConn1 -- Orifice Release/LConn2

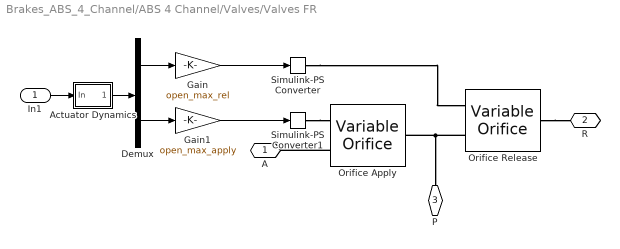
== system Brakes_ABS_4_Channel/ABS 4 Channel/Valves/Valves FR ==
  In1 : Inport
  Actuator Dynamics : Subsystem  mask(First-order lag supporting vector signals){b=brkTs, x_initial=0}
      mask prompts: b "Filter time constant"; x_initial "Initial output"
      mask help: Models a lag of the form 1/(b*s+1) where s is the Laplace operator.
  Demux : Demux  Outputs=2
  Gain : Gain  Gain=open_max_rel
      settings: AttributesFormatString=%<Gain>
  Gain1 : Gain  Gain=open_max_apply
      settings: AttributesFormatString=%<Gain>
  Orifice Apply : sh_lib/Orifices/Variable Orifice  mdl_type=1  area_max=area_max_apply m^2  opening_max=open_max_apply m  opening_tab=[-.002, 0, .002, .005, .015] m  area_tab=[1e-09, 2.0352e-07, 4.0736e-05, .00011438, .00034356] m^2  pressure_tab=[-10000000, -5000000, -2000000, 2000000, 5000000, 10000000] Pa  flow_rate_tab=[-1e-07, -7.0711e-08, -4.4721e-08, 4.4721e-08, 7.0711e-08, 1e-07; -2.0352e-05, -1.4391e-05, -9.1017e-06, 9.1017e-06, 1.4391e-05, 2.0352e-05; -.0040736, -.0028805, -.0018218, .0018218, .0028805, .0040736; -.011438, -.0080879, -.0051152, .0051152, .0080879, .011438; -.034356, -.024293, -.015364, .015364, .024293, .034356] m^3/s  interp_method=1  extrap_method=1  or=1  C_d=0.7  x_0=0 m  A_leak=1e-12 m^2  lam_spec=1  B_lam=0.999  Re_cr=12  flow_rate_specify=off  flow_rate_priority=None  flow_rate=0 m^3/s  flow_rate_nominal_specify=off  flow_rate_nominal_unit=m^3/s  flow_rate_nominal_value=1  pressure_drop_specify=off  pressure_drop_priority=None  pressure_drop=0 Pa  pressure_drop_nominal_specify=off  pressure_drop_nominal_unit=Pa  pressure_drop_nominal_value=1
      settings: SourceProductName=Simscape Fluids  SourceProductBaseCode=SH  InternalSimscapePortConfiguration="{\"Bottom\":[],\"Left\":[{\"id\":\"S\",\"label\":\"S\",\"type\":\"input\"},{\"id\":\"A\",\"label\":\"A\",\"type\":\"foundation.hydraulic.hydraulic\"}],\"Right\":[{\"id\":\"B\",\"label\":\"B\",\"type\":\"foundation.hydraulic.hydraulic\"}],\"Top\":[]}"
  Orifice Release : sh_lib/Orifices/Variable Orifice  mdl_type=1  area_max=area_max_rel m^2  opening_max=open_max_rel m  opening_tab=[-.002, 0, .002, .005, .015] m  area_tab=[1e-09, 2.0352e-07, 4.0736e-05, .00011438, .00034356] m^2  pressure_tab=[-10000000, -5000000, -2000000, 2000000, 5000000, 10000000] Pa  flow_rate_tab=[-1e-07, -7.0711e-08, -4.4721e-08, 4.4721e-08, 7.0711e-08, 1e-07; -2.0352e-05, -1.4391e-05, -9.1017e-06, 9.1017e-06, 1.4391e-05, 2.0352e-05; -.0040736, -.0028805, -.0018218, .0018218, .0028805, .0040736; -.011438, -.0080879, -.0051152, .0051152, .0080879, .011438; -.034356, -.024293, -.015364, .015364, .024293, .034356] m^3/s  interp_method=1  extrap_method=1  or=1  C_d=0.7  x_0=0 m  A_leak=1e-12 m^2  lam_spec=1  B_lam=0.999  Re_cr=12  flow_rate_specify=off  flow_rate_priority=None  flow_rate=0 m^3/s  flow_rate_nominal_specify=off  flow_rate_nominal_unit=m^3/s  flow_rate_nominal_value=1  pressure_drop_specify=off  pressure_drop_priority=None  pressure_drop=0 Pa  pressure_drop_nominal_specify=off  pressure_drop_nominal_unit=Pa  pressure_drop_nominal_value=1
      settings: SourceProductName=Simscape Fluids  SourceProductBaseCode=SH  InternalSimscapePortConfiguration="{\"Bottom\":[],\"Left\":[{\"id\":\"S\",\"label\":\"S\",\"type\":\"input\"},{\"id\":\"A\",\"label\":\"A\",\"type\":\"foundation.hydraulic.hydraulic\"}],\"Right\":[{\"id\":\"B\",\"label\":\"B\",\"type\":\"foundation.hydraulic.hydraulic\"}],\"Top\":[]}"
  Simulink-PS Converter : nesl_utility/Simulink-PS Converter  PhysicalDomain=network_engine_domain  SubClassName=ps_input  LeftPortType=input  RightPortType=output  PseudoPeriodic=off  Frequencies=[]  NoiseDistribution=none  NoiseParameters=[]  Unit=1  AffineConversion=off  FilteringAndDerivatives=provide  SimscapeFilterOrder=1  InputFilterTimeConstant=0.001  UdotUserProvided=0
  Simulink-PS Converter1 : nesl_utility/Simulink-PS Converter  PhysicalDomain=network_engine_domain  SubClassName=ps_input  LeftPortType=input  RightPortType=output  PseudoPeriodic=off  Frequencies=[]  NoiseDistribution=none  NoiseParameters=[]  Unit=1  AffineConversion=off  FilteringAndDerivatives=provide  SimscapeFilterOrder=1  InputFilterTimeConstant=0.001  UdotUserProvided=0
  A : PMIOPort  Side=Left
  R : PMIOPort  Port=2  Side=Left
  P : PMIOPort  Port=3  Side=Right
  wires:
  Actuator Dynamics/1(Out) -> Demux/1
  In1/1 -> Actuator Dynamics/1(In)
  Demux/1 -> Gain/1
  Gain/1 -> Simulink-PS Converter/1
  Gain1/1 -> Simulink-PS Converter1/1
  Demux/2 -> Gain1/1
  connections:
  Orifice Release/LConn2 -- Orifice Apply/RConn1 -- P/RConn1
  Orifice Release/RConn1 -- R/RConn1
  Simulink-PS Converter/RConn1 -- Orifice Release/LConn1
  Simulink-PS Converter1/RConn1 -- Orifice Apply/LConn1
  Orifice Apply/LConn2 -- A/RConn1

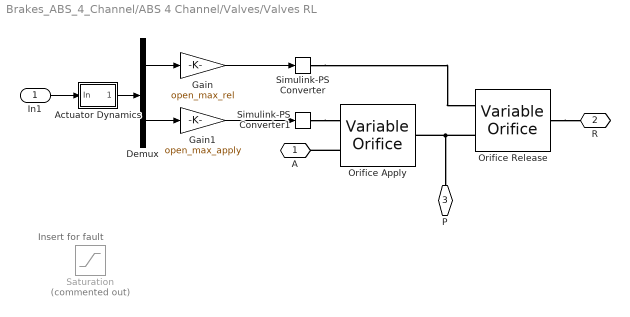
== system Brakes_ABS_4_Channel/ABS 4 Channel/Valves/Valves RL ==
  note: Insert for fault
  In1 : Inport
  Actuator Dynamics : Subsystem  mask(First-order lag supporting vector signals){b=brkTs, x_initial=0}
      mask prompts: b "Filter time constant"; x_initial "Initial output"
      mask help: Models a lag of the form 1/(b*s+1) where s is the Laplace operator.
  Demux : Demux  Outputs=2
  Gain : Gain  Gain=open_max_rel
      settings: AttributesFormatString=%<Gain>
  Gain1 : Gain  Gain=open_max_apply
      settings: AttributesFormatString=%<Gain>
  Orifice Apply : sh_lib/Orifices/Variable Orifice  mdl_type=1  area_max=area_max_apply m^2  opening_max=open_max_apply m  opening_tab=[-.002, 0, .002, .005, .015] m  area_tab=[1e-09, 2.0352e-07, 4.0736e-05, .00011438, .00034356] m^2  pressure_tab=[-10000000, -5000000, -2000000, 2000000, 5000000, 10000000] Pa  flow_rate_tab=[-1e-07, -7.0711e-08, -4.4721e-08, 4.4721e-08, 7.0711e-08, 1e-07; -2.0352e-05, -1.4391e-05, -9.1017e-06, 9.1017e-06, 1.4391e-05, 2.0352e-05; -.0040736, -.0028805, -.0018218, .0018218, .0028805, .0040736; -.011438, -.0080879, -.0051152, .0051152, .0080879, .011438; -.034356, -.024293, -.015364, .015364, .024293, .034356] m^3/s  interp_method=1  extrap_method=1  or=1  C_d=0.7  x_0=0 m  A_leak=1e-12 m^2  lam_spec=1  B_lam=0.999  Re_cr=12  flow_rate_specify=off  flow_rate_priority=None  flow_rate=0 m^3/s  flow_rate_nominal_specify=off  flow_rate_nominal_unit=m^3/s  flow_rate_nominal_value=1  pressure_drop_specify=off  pressure_drop_priority=None  pressure_drop=0 Pa  pressure_drop_nominal_specify=off  pressure_drop_nominal_unit=Pa  pressure_drop_nominal_value=1
      settings: SourceProductName=Simscape Fluids  SourceProductBaseCode=SH  InternalSimscapePortConfiguration="{\"Bottom\":[],\"Left\":[{\"id\":\"S\",\"label\":\"S\",\"type\":\"input\"},{\"id\":\"A\",\"label\":\"A\",\"type\":\"foundation.hydraulic.hydraulic\"}],\"Right\":[{\"id\":\"B\",\"label\":\"B\",\"type\":\"foundation.hydraulic.hydraulic\"}],\"Top\":[]}"
  Orifice Release : sh_lib/Orifices/Variable Orifice  mdl_type=1  area_max=area_max_rel m^2  opening_max=open_max_rel m  opening_tab=[-.002, 0, .002, .005, .015] m  area_tab=[1e-09, 2.0352e-07, 4.0736e-05, .00011438, .00034356] m^2  pressure_tab=[-10000000, -5000000, -2000000, 2000000, 5000000, 10000000] Pa  flow_rate_tab=[-1e-07, -7.0711e-08, -4.4721e-08, 4.4721e-08, 7.0711e-08, 1e-07; -2.0352e-05, -1.4391e-05, -9.1017e-06, 9.1017e-06, 1.4391e-05, 2.0352e-05; -.0040736, -.0028805, -.0018218, .0018218, .0028805, .0040736; -.011438, -.0080879, -.0051152, .0051152, .0080879, .011438; -.034356, -.024293, -.015364, .015364, .024293, .034356] m^3/s  interp_method=1  extrap_method=1  or=1  C_d=0.7  x_0=0 m  A_leak=1e-12 m^2  lam_spec=1  B_lam=0.999  Re_cr=12  flow_rate_specify=off  flow_rate_priority=None  flow_rate=0 m^3/s  flow_rate_nominal_specify=off  flow_rate_nominal_unit=m^3/s  flow_rate_nominal_value=1  pressure_drop_specify=off  pressure_drop_priority=None  pressure_drop=0 Pa  pressure_drop_nominal_specify=off  pressure_drop_nominal_unit=Pa  pressure_drop_nominal_value=1
      settings: SourceProductName=Simscape Fluids  SourceProductBaseCode=SH  InternalSimscapePortConfiguration="{\"Bottom\":[],\"Left\":[{\"id\":\"S\",\"label\":\"S\",\"type\":\"input\"},{\"id\":\"A\",\"label\":\"A\",\"type\":\"foundation.hydraulic.hydraulic\"}],\"Right\":[{\"id\":\"B\",\"label\":\"B\",\"type\":\"foundation.hydraulic.hydraulic\"}],\"Top\":[]}"
  Saturation : Saturate  Commented=on  UpperLimit=inf  LowerLimit=0.5
  Simulink-PS Converter : nesl_utility/Simulink-PS Converter  PhysicalDomain=network_engine_domain  SubClassName=ps_input  LeftPortType=input  RightPortType=output  PseudoPeriodic=off  Frequencies=[]  NoiseDistribution=none  NoiseParameters=[]  Unit=1  AffineConversion=off  FilteringAndDerivatives=provide  SimscapeFilterOrder=1  InputFilterTimeConstant=0.001  UdotUserProvided=0
  Simulink-PS Converter1 : nesl_utility/Simulink-PS Converter  PhysicalDomain=network_engine_domain  SubClassName=ps_input  LeftPortType=input  RightPortType=output  PseudoPeriodic=off  Frequencies=[]  NoiseDistribution=none  NoiseParameters=[]  Unit=1  AffineConversion=off  FilteringAndDerivatives=provide  SimscapeFilterOrder=1  InputFilterTimeConstant=0.001  UdotUserProvided=0
  A : PMIOPort  Side=Left
  R : PMIOPort  Port=2  Side=Left
  P : PMIOPort  Port=3  Side=Right
  wires:
  In1/1 -> Actuator Dynamics/1(In)
  Actuator Dynamics/1(Out) -> Demux/1
  Demux/1 -> Gain/1
  Gain/1 -> Simulink-PS Converter/1
  Gain1/1 -> Simulink-PS Converter1/1
  Demux/2 -> Gain1/1
  connections:
  Orifice Release/LConn2 -- Orifice Apply/RConn1 -- P/RConn1
  Orifice Release/RConn1 -- R/RConn1
  Simulink-PS Converter/RConn1 -- Orifice Release/LConn1
  Simulink-PS Converter1/RConn1 -- Orifice Apply/LConn1
  Orifice Apply/LConn2 -- A/RConn1
